simulink model "IncrementalConductanceSim"  (R2020b)
settings: Solver=VariableStepAuto  StartTime=0.0  StopTime=10.0  RelTol=1e-3
libraries: powerlib x10, re_lib x1, powerlib_meascontrol x1
settings Model: Creator=Hannah  LastModifiedBy=Hannah

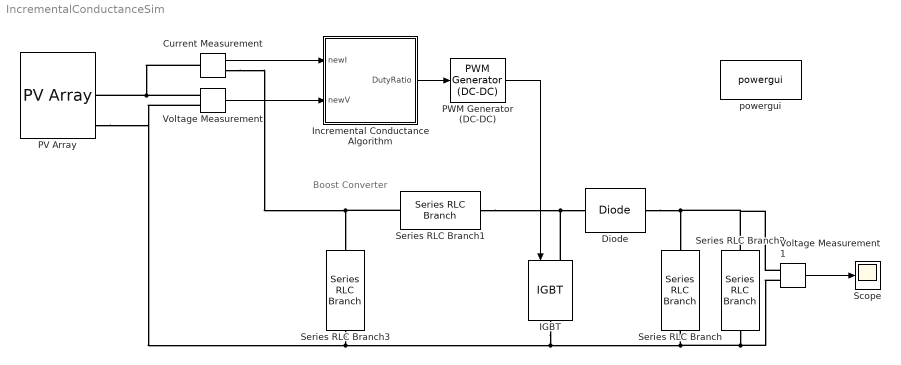
== system IncrementalConductanceSim ==
  note: Boost Converter
  Current Measurement : powerlib/Measurements/Current Measurement  PhasorSimulation=off  OutputType=Complex  PSBequivalent=0
  Diode : powerlib/Power Electronics/Diode  Ron=0.001  Lon=0  Vf=0.8  IC=0  UseSnubber=0  Rs=500  Cs=250e-9  Measurements=off
  IGBT : powerlib/Power Electronics/IGBT  Ron=0.001  Lon=0  Vf=1  Tf=1e-6  Tt=2e-6  IC=0  Rs=1e5  Cs=inf  Measurements=off
  Incremental Conductance Algorithm : Subsystem
  PV Array : re_lib/Solar/PV Array  Npar=40  Nser=10  PlotType=array @ 1000 W/m2 & specified temperatures  S_vec="[ 1000  500  100 ]"  Temp_C_vec="[ 45 25  ]"  ModuleName=User-defined  PlotWhenSelected=off  Pm=213.15  Ncell=60  Voc=36.3  Isc=7.84  Vm=29  Im=7.35  beta_Voc_pc=-0.36099  alpha_Isc_pc=0.102  beta_Voc=-0.13104  alpha_Isc=0.0079968  IL=7.8654  I0=2.9273e-10  nI=0.98119  Rsh=313.0553  Rs=0.39381  RobustModel=off  RobustCellTemperature=313.3991  BAL=on  Tc=1e-6  Tfilter=5e-5
  PWM Generator (DC-DC) : powerlib_meascontrol/Pulse & Signal Generators/PWM Generator (DC-DC)  Fsw=5000  Ts=0
  Scope : Scope
  Series RLC Branch : powerlib/Elements/Series RLC Branch  LConnTagsString=__new0  RConnTagsString=__new0  BranchType=C  Resistance=1  Inductance=1e-3  SetiL0=off  InitialCurrent=0  Capacitance=1e-6  Setx0=off  InitialVoltage=0  Measurements=None
  Series RLC Branch1 : powerlib/Elements/Series RLC Branch  LConnTagsString=__new0  RConnTagsString=__new0  BranchType=RL  Resistance=1  Inductance=1e-3  SetiL0=off  InitialCurrent=0  Capacitance=1e-6  Setx0=off  InitialVoltage=0  Measurements=None
  Series RLC Branch2 : powerlib/Elements/Series RLC Branch  LConnTagsString=__new0  RConnTagsString=__new0  BranchType=R  Resistance=1  Inductance=1e-3  SetiL0=off  InitialCurrent=0  Capacitance=1e-6  Setx0=off  InitialVoltage=0  Measurements=None
  Series RLC Branch3 : powerlib/Elements/Series RLC Branch  LConnTagsString=__new0  RConnTagsString=__new0  BranchType=C  Resistance=1  Inductance=1e-3  SetiL0=off  InitialCurrent=0  Capacitance=1e-6  Setx0=off  InitialVoltage=0  Measurements=None
  Voltage Measurement : powerlib/Measurements/Voltage Measurement  PhasorSimulation=off  OutputType=Complex  PSBequivalent=0
  Voltage Measurement1 : powerlib/Measurements/Voltage Measurement  PhasorSimulation=off  OutputType=Complex  PSBequivalent=0
  powergui : powerlib/powergui  Priority=1  SimulationMode=Discrete  SampleTime=1e-06  frequency=60  Iterations=50  frequencyindice=60  Pbase=100e6  ErrMax=1e-4  UnitsV=kV  UnitsW=MW  buscounter=0  FunctionMessages=off  echomessages=off  EnableUseOfTLC=off  CurrentSourceSwitches=off  DisableSnubberDevices=off  DisableRonSwitches=off  DisableVfSwitches=off  DisplayEquations=off  AutomaticDiscreteSolvers=off  SolverType=Tustin/Backward Euler (TBE)  Interpol=off  ExternalGateDelay=off  methode=off  Ts=100  x0status=blocks  SPID=on  SwTol=0  HookPort=off  NonlinearTolerance=1e-4  nMaxIteration=100  ContinueOnMaxIteration=off  RestoreLinks=warning  ResistiveCurrentMeasurement=off  Frange=[0:2:500]  Ylog=off  Xlog=on  ShowGrid=off  save=off  variable=ZData  structure=0  ZoomFFT=off  StartTime=0.0  cycles=1  DisplayStyle=1  fundamental=60  FreqAxis=off  MaxFrequency=1000  frequencyindicesteady=1  RmsSteady=1  display=off
  wires:
  Incremental Conductance Algorithm/1(DutyRatio) -> PWM Generator (DC-DC)/1
  Voltage Measurement/1 -> Incremental Conductance Algorithm/2(newV)
  Current Measurement/1 -> Incremental Conductance Algorithm/1(newI)
  PWM Generator (DC-DC)/1 -> IGBT/1
  Voltage Measurement1/1 -> Scope/1
  connections:
  Voltage Measurement/LConn1 -- Current Measurement/LConn1 -- PV Array/RConn1
  IGBT/LConn1 -- Diode/LConn1 -- Series RLC Branch1/RConn1
  Diode/RConn1 -- Voltage Measurement1/LConn1 -- Series RLC Branch2/LConn1 -- Series RLC Branch/LConn1
  Series RLC Branch2/RConn1 -- Voltage Measurement/LConn2 -- PV Array/RConn2 -- Series RLC Branch3/RConn1 -- IGBT/RConn1 -- Series RLC Branch/RConn1 -- Voltage Measurement1/LConn2
  Series RLC Branch1/LConn1 -- Current Measurement/RConn1 -- Series RLC Branch3/LConn1

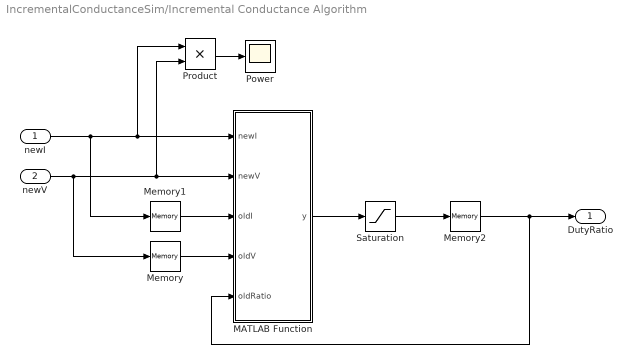
== system IncrementalConductanceSim/Incremental Conductance Algorithm ==
  newI : Inport
  newV : Inport  Port=2
  MATLAB Function : MATLAB Function  TreatAsAtomicUnit=on
  Memory : Memory
  Memory1 : Memory
  Memory2 : Memory
  Power : Scope
  Product : Product
  Saturation : Saturate  UpperLimit=0.9  LowerLimit=0
  DutyRatio : Outport
  wires:
  newI/1 -> Product/1, MATLAB Function/1(newI), Memory1/1
  Memory2/1 -> DutyRatio/1, MATLAB Function/5(oldRatio)
  Memory/1 -> MATLAB Function/4(oldV)
  Saturation/1 -> Memory2/1
  MATLAB Function/1(y) -> Saturation/1
  Memory1/1 -> MATLAB Function/3(oldI)
  newV/1 -> Product/2, MATLAB Function/2(newV), Memory/1
  Product/1 -> Power/1

== matlab function IncrementalConductanceSim/Incremental Conductance Algorithm/MATLAB Function ==
  data: newI input; newV input; oldI input; y output; oldV input; oldRatio input
function y = fcn(newI, newV, oldI, oldV, oldRatio)
    dutyRatio = 0.5;
    change = 0.00005;
    
    deltaV = newV - oldV; %find change in voltage
    deltaI = newI - oldI; %find change in current
    
    if(deltaV == 0) 
        if(deltaI == 0)
            dutyRatio = oldRatio;
        else
            if(deltaI > 0)
                dutyRatio = oldRatio + change; %increase duty ratio
            else
                dutyRatio = oldRatio - change; %decrease duty ratio
            end
        end
    else
        if(deltaI/deltaV == -(newI/newV))
            dutyRatio = oldRatio; %no change
        else
            if(deltaI/deltaV > -(newI/newV))
                dutyRatio = oldRatio + change; %increase duty ratio
            else
                dutyRatio = oldRatio - change; %decrease duty ratio
            end
        end
    end
y = dutyRatio;
